simulink library "Conducteur"  (R2018a)
settings: Solver=VariableStepAuto  StartTime=0.0  StopTime=10.0  RelTol=1e-3
values from neighbouring files (symbols this model uses):
  c_dist_int = (0:1:1999)    [UntitFSDAFled.m]
  vlim = 0    [LimitationVitesse.m]    (also in getMaxSpeed.m; getMaxSpeed2.m)
undefined symbols (not defined in the file or in its folder): dist_tot_int
libraries: simulink x3
settings Model: Creator=thomas.moser  LastModifiedBy=thomas.moser

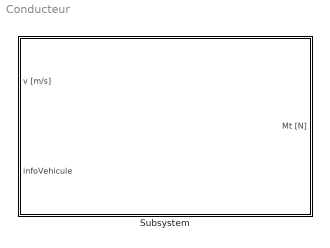
== system Conducteur ==
  Subsystem : Subsystem

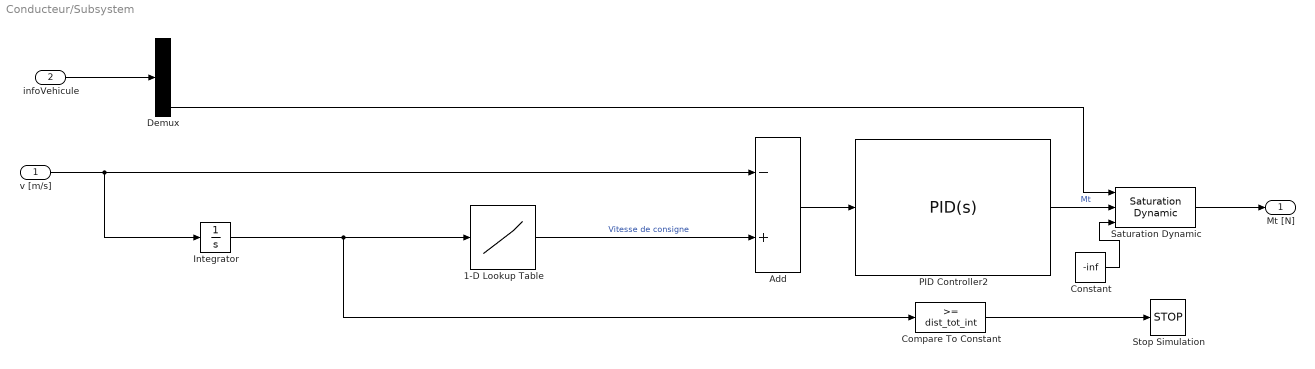
== system Conducteur/Subsystem ==
  v [m/s] : Inport
  infoVehicule : Inport  Port=2
  1-D Lookup Table : Lookup_n-D  NumberOfTableDimensions=1  BreakpointsForDimension1=c_dist_int  Table=vlim  InternalRulePriority=Speed  RndMeth=Simplest  InputSameDT=on
  Add : Sum  Inputs=-+
  Compare To Constant : simulink/Logic and Bit Operations/Compare To Constant  relop=>=  const=dist_tot_int  OutDataTypeStr=boolean
  Constant : Constant  Value=-inf
  Demux : Demux  Outputs=5
  Integrator : Integrator
  PID Controller2 : simulink/Continuous/PID Controller  Controller=PID  TimeDomain=Continuous-time  SampleTime=-1  IntegratorMethod=Forward Euler  FilterMethod=Forward Euler  Form=Parallel  UseFilter=on  ControllerParametersSource=internal  P=2000  I=10  D=0  N=200  InitialConditionSource=internal  InitialConditionForIntegrator=0  InitialConditionForFilter=0  ExternalReset=none  LimitOutput=off  UpperSaturationLimit=inf  LowerSaturationLimit=-inf  LinearizeAsGain=on  AntiWindupMode=none  Kb=1  TrackingMode=off  Kt=1  PParamMin=[]  PParamMax=[]  IParamMin=[]  IParamMax=[]  DParamMin=[]  DParamMax=[]  NParamMin=[]  NParamMax=[]  KbParamMin=[]  KbParamMax=[]  KtParamMin=[]  KtParamMax=[]  POutMin=[]  POutMax=[]  IOutMin=[]  IOutMax=[]  DOutMin=[]  DOutMax=[]  NOutMin=[]  NOutMax=[]  KbOutMin=[]  KbOutMax=[]  KtOutMin=[]  KtOutMax=[]  IntegratorOutMin=[]  IntegratorOutMax=[]  FilterOutMin=[]  FilterOutMax=[]  SumOutMin=[]  SumOutMax=[]  SumI1OutMin=[]  SumI1OutMax=[]  SumI2OutMin=[]  SumI2OutMax=[]  SumI3OutMin=[]  SumI3OutMax=[]  SumDOutMin=[]  SumDOutMax=[]  SaturationOutMin=[]  SaturationOutMax=[]  IntegratorContinuousStateAttributes=''  IntegratorStateMustResolveToSignalObject=off  IntegratorRTWStateStorageClass=Auto  FilterContinuousStateAttributes=''  FilterStateMustResolveToSignalObject=off  FilterRTWStateStorageClass=Auto  DifferentiatorICPrevScaledInput=0  DifferentiatorOutMin=[]  DifferentiatorOutMax=[]  FilterDiffOutCoefMin=[]  FilterDiffOutCoefMax=[]  SumDenOutMin=[]  SumDenOutMax=[]  SumNumOutMin=[]  SumNumOutMax=[]  ReciprocalOutMin=[]  ReciprocalOutMax=[]  DivideOutMin=[]  DivideOutMax=[]  TunerSelectOption=Frequency Response Based
  Saturation Dynamic : simulink/Discontinuities/Saturation Dynamic  OutMin=[]  OutMax=[]  OutDataTypeStr=Inherit: Same as second input  OutDataType=fixdt(1, 16)  OutScaling=2^-10  DoSatur=off
  Stop Simulation : Stop
  Mt [N] : Outport
  wires:
  Add/1 -> PID Controller2/1
  Compare To Constant/1 -> Stop Simulation/1
  Integrator/1 -> Compare To Constant/1, 1-D Lookup Table/1
  PID Controller2/1 -> Saturation Dynamic/2  "Mt"
  1-D Lookup Table/1 -> Add/2  "Vitesse de consigne"
  v [m/s]/1 -> Integrator/1, Add/1
  infoVehicule/1 -> Demux/1
  Demux/5 -> Saturation Dynamic/1
  Saturation Dynamic/1 -> Mt [N]/1
  Constant/1 -> Saturation Dynamic/3
